simulink model "testJointMuxDemux"  (R2016b)
settings: Solver=ode4  StartTime=0.0  StopTime=inf  FixedStep=0.002  RelTol=1e-3  EnableMultiTasking=on
libraries: VariousLibrary x6, slrtlib x1
settings Model: SimulationMode=external  Creator=march  LastModifiedBy=march
settings SolverCC: EnableConcurrentExecution=on
settings DataIOCC: SaveFormat=StructureWithTime
settings OptimizationCC: BlockReduction=off  OptimizeBlockIOStorage=off  BufferReuse=off  GlobalBufferReuse=off  ExpressionFolding=off  LocalBlockOutputs=off
settings HardwareCC: ProdBitPerPointer=32  ProdBitPerSizeT=32  ProdBitPerPtrDiffT=32  ProdLargestAtomicFloat=None  ProdWordSize=32  ProdLongLongMode=on  ProdHWDeviceType=Generic->32-bit x86 compatible
settings RTWCC: SystemTargetFile=slrt.tlc  TemplateMakefile=slrt_default_tmf  Description=Simulink Real-Time  RTWCompilerOptimization=on

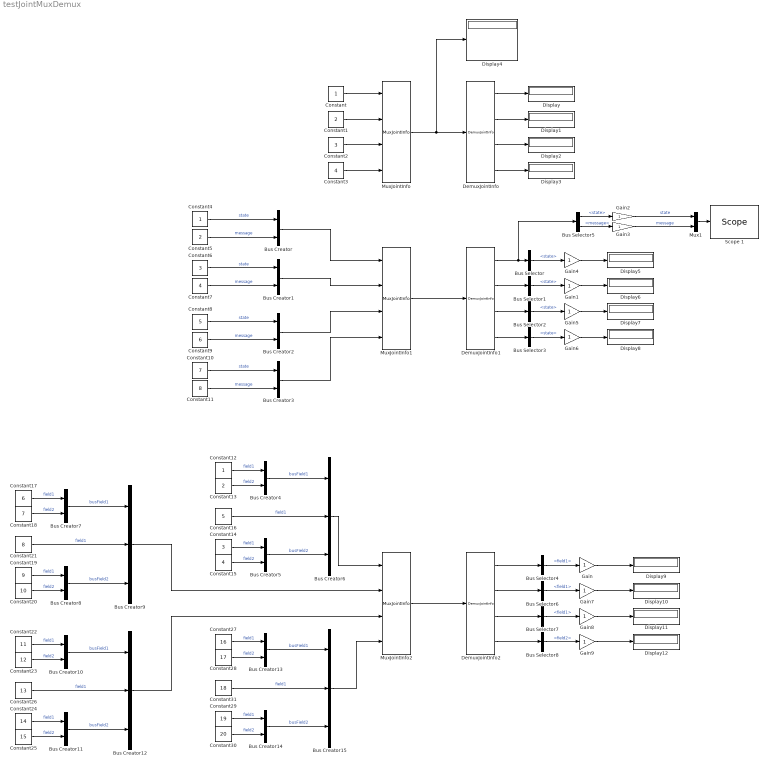
== system testJointMuxDemux ==
  Bus Creator{,1..3} (4 alike) : BusCreator  Inputs=2  OutDataTypeStr=Bus: EtherCATSendToInputDevice  NonVirtualBus=on
  Bus Creator{4..5,7..8,10..11,13..14} (8 alike) : BusCreator  Inputs=2  OutDataTypeStr=Bus: TestBusElement  NonVirtualBus=on
  Bus Creator{6,9,12,15} (4 alike) : BusCreator  Inputs=3  OutDataTypeStr=Bus: TestBusBus  NonVirtualBus=on
  Bus Selector{,1..3} (4 alike) : BusSelector  OutputSignals=state
  Bus Selector4 : BusSelector  OutputSignals=field1
  Bus Selector5 : BusSelector  OutputSignals=state,message
  Bus Selector6 : BusSelector  OutputSignals=busField1.field1
  Bus Selector7 : BusSelector  OutputSignals=busField2.field1
  Bus Selector8 : BusSelector  OutputSignals=busField2.field2
  Constant : Constant
  Constant1 : Constant  Value=2
  Constant10 : Constant  Value=7
  Constant11 : Constant  Value=8
  Constant12 : Constant
  Constant13 : Constant  Value=2
  Constant14 : Constant  Value=3
  Constant15 : Constant  Value=4
  Constant16 : Constant  Value=5  OutDataTypeStr=double
  Constant17 : Constant  Value=6
  Constant18 : Constant  Value=7
  Constant19 : Constant  Value=9
  Constant2 : Constant  Value=3
  Constant20 : Constant  Value=10
  Constant21 : Constant  Value=8  OutDataTypeStr=double
  Constant22 : Constant  Value=11
  Constant23 : Constant  Value=12
  Constant24 : Constant  Value=14
  Constant25 : Constant  Value=15
  Constant26 : Constant  Value=13  OutDataTypeStr=double
  Constant27 : Constant  Value=16
  Constant28 : Constant  Value=17
  Constant29 : Constant  Value=19
  Constant3 : Constant  Value=4
  Constant30 : Constant  Value=20
  Constant31 : Constant  Value=18  OutDataTypeStr=double
  Constant4 : Constant
  Constant5 : Constant  Value=2
  Constant6 : Constant  Value=3
  Constant7 : Constant  Value=4
  Constant8 : Constant  Value=5
  Constant9 : Constant  Value=6
  DemuxJointInfo : VariousLibrary/DemuxJointInfo
  DemuxJointInfo1 : VariousLibrary/DemuxJointInfo
  DemuxJointInfo2 : VariousLibrary/DemuxJointInfo
  Display{,1..12} (13 alike) : Display
  Gain{,1..9} (10 alike) : Gain
  Mux1 : Mux  Inputs=2
  MuxJointInfo : VariousLibrary/MuxJointInfo
  MuxJointInfo1 : VariousLibrary/MuxJointInfo
  MuxJointInfo2 : VariousLibrary/MuxJointInfo
  Scope 1 : slrtlib/Displays and Logging/Scope   scopeno=1  scopetype=Target  autostart=on  viewmode=Numerical  formatstr='%15.6f'  grid=on  ylimits=[0,0]  nosamples=250  noprepostsamples=0  interleave=1  triggermode=FreeRun  triggersignal=1  trigsignalfromport=off  triggerlevel=0.0  triggerslope=Either  triggerscope=1  triggersample=0  filename=data.dat  mode=Lazy  writesize=512  autorestart=off  dynamicfilemode=off  maxwritefilesize=512*1024^2
  wires:
  Constant/1 -> MuxJointInfo/1
  Constant1/1 -> MuxJointInfo/2
  Constant2/1 -> MuxJointInfo/3
  Constant3/1 -> MuxJointInfo/4
  MuxJointInfo/1 -> Display4/1, DemuxJointInfo/1
  DemuxJointInfo/1 -> Display/1
  DemuxJointInfo/2 -> Display1/1
  DemuxJointInfo/3 -> Display2/1
  DemuxJointInfo/4 -> Display3/1
  Constant5/1 -> Bus Creator/2  "message"
  Constant4/1 -> Bus Creator/1  "state"
  Constant7/1 -> Bus Creator1/2  "message"
  Constant6/1 -> Bus Creator1/1  "state"
  Constant9/1 -> Bus Creator2/2  "message"
  Constant8/1 -> Bus Creator2/1  "state"
  Constant11/1 -> Bus Creator3/2  "message"
  Constant10/1 -> Bus Creator3/1  "state"
  Bus Creator/1 -> MuxJointInfo1/1
  Bus Creator1/1 -> MuxJointInfo1/2
  Bus Creator2/1 -> MuxJointInfo1/3
  Bus Creator3/1 -> MuxJointInfo1/4
  MuxJointInfo1/1 -> DemuxJointInfo1/1
  DemuxJointInfo1/1 -> Bus Selector5/1, Bus Selector/1
  DemuxJointInfo1/4 -> Bus Selector3/1
  DemuxJointInfo1/3 -> Bus Selector2/1
  DemuxJointInfo1/2 -> Bus Selector1/1
  Bus Selector/1 -> Gain4/1  "<state>"
  Bus Selector5/1 -> Gain2/1  "<state>"
  Bus Selector5/2 -> Gain3/1  "<message>"
  Gain3/1 -> Mux1/2  "message"
  Gain2/1 -> Mux1/1  "state"
  Mux1/1 -> Scope 1/1
  Gain4/1 -> Display5/1
  Bus Selector1/1 -> Gain1/1  "<state>"
  Bus Selector2/1 -> Gain5/1  "<state>"
  Bus Selector3/1 -> Gain6/1  "<state>"
  Gain1/1 -> Display6/1
  Gain5/1 -> Display7/1
  Gain6/1 -> Display8/1
  MuxJointInfo2/1 -> DemuxJointInfo2/1
  Constant12/1 -> Bus Creator4/1  "field1"
  Constant13/1 -> Bus Creator4/2  "field2"
  Constant14/1 -> Bus Creator5/1  "field1"
  Constant15/1 -> Bus Creator5/2  "field2"
  Bus Creator4/1 -> Bus Creator6/1  "busField1"
  Bus Creator6/1 -> MuxJointInfo2/1
  DemuxJointInfo2/1 -> Bus Selector4/1
  DemuxJointInfo2/2 -> Bus Selector6/1
  DemuxJointInfo2/3 -> Bus Selector7/1
  DemuxJointInfo2/4 -> Bus Selector8/1
  Bus Selector4/1 -> Gain/1  "<field1>"
  Bus Selector6/1 -> Gain7/1  "<field1>"
  Bus Selector7/1 -> Gain8/1  "<field1>"
  Bus Selector8/1 -> Gain9/1  "<field2>"
  Gain/1 -> Display9/1
  Gain7/1 -> Display10/1
  Gain8/1 -> Display11/1
  Gain9/1 -> Display12/1
  Constant16/1 -> Bus Creator6/2  "field1"
  Bus Creator5/1 -> Bus Creator6/3  "busField2"
  Constant17/1 -> Bus Creator7/1  "field1"
  Constant18/1 -> Bus Creator7/2  "field2"
  Constant19/1 -> Bus Creator8/1  "field1"
  Constant20/1 -> Bus Creator8/2  "field2"
  Bus Creator7/1 -> Bus Creator9/1  "busField1"
  Constant21/1 -> Bus Creator9/2  "field1"
  Bus Creator8/1 -> Bus Creator9/3  "busField2"
  Constant22/1 -> Bus Creator10/1  "field1"
  Constant23/1 -> Bus Creator10/2  "field2"
  Constant24/1 -> Bus Creator11/1  "field1"
  Constant25/1 -> Bus Creator11/2  "field2"
  Bus Creator10/1 -> Bus Creator12/1  "busField1"
  Constant26/1 -> Bus Creator12/2  "field1"
  Bus Creator11/1 -> Bus Creator12/3  "busField2"
  Constant27/1 -> Bus Creator13/1  "field1"
  Constant28/1 -> Bus Creator13/2  "field2"
  Constant29/1 -> Bus Creator14/1  "field1"
  Constant30/1 -> Bus Creator14/2  "field2"
  Bus Creator13/1 -> Bus Creator15/1  "busField1"
  Constant31/1 -> Bus Creator15/2  "field1"
  Bus Creator14/1 -> Bus Creator15/3  "busField2"
  Bus Creator9/1 -> MuxJointInfo2/2
  Bus Creator12/1 -> MuxJointInfo2/3
  Bus Creator15/1 -> MuxJointInfo2/4
